simulink model "rocketmodel"  (R2019b)
settings: Solver=VariableStepAuto  StartTime=0.0  StopTime=1  RelTol=1e-3
values from neighbouring files (symbols this model uses):
  g = 9.8    [main_rocketmodel.m]    (also in main_sim_rocket.m; rocket_model.m; sim_lin.m; test_bangbang.m)
  gimbal_eq = 0    [main_rocketmodel.m]    (also in main_sim_rocket.m; sim_lin.m)
  J_T = 40267    [main_rocketmodel.m]    (also in main_sim_rocket.m; rocket_model.m = 10)
  K = minreal(Q/(1+Q*P))    [cost.m]    (also in cost_LQ.m = tf((conv(denQ{1},numK0{1})+conv(numQ{1},den_sys{1})),(conv(d; cost_con.m = tf((conv(denQ{1},numK0{1})+conv(numQ{1},den_sys{1})),(conv(d; cost_disturb.m = tf((conv(denQ{1},numK0{1})+conv(numQ{1},den_sys{1})),(conv(d; fminunc_LQ.m = tf((conv(denQ{1},numK0{1})+conv(numQ{1},den_sys{1})),(conv(d)
  K_2 = (tf((conv(denQ{1},num{1})+conv(numQ{1},den_sys{1})),(conv(denQ{1},den{1})-conv(numQ{1},num_sys{1}))))    [test.m]    (also in test_qvalues.m = Q_2/(1+Q_2*P))
  m = 549054    [main_rocketmodel.m]    (also in main_sim_rocket.m; rocket_model.m = 25.4; sim_lin.m; test_bangbang.m)
  sys = ss(A,B,C,D)    [controller_design.m]    (also in main_yp_fminunc.m; rocket_controllerdesign.m; rocket_controllerdesign_z.m; rocket_model.m)
  t_on = 14.6    [main_rocketmodel.m]    (also in main_sim_rocket.m; test_bangbang.m)
  Ts = 0.001    [main_rocketmodel.m]    (also in main_sim_rocket.m; sim_lin.m; square_sig.m; sum_squares_sig.m)
  x_0 = 0    [main_rocketmodel.m]    (also in main_sim_rocket.m)
  z_0 = 4000    [main_rocketmodel.m]    (also in main_sim_rocket.m; sim_lin.m; test_bangbang.m)
libraries: simulink x1
settings Model: Creator=bia  LastModifiedBy=bia
settings DataIOCC: ExternalInput=[t, Fe]  SignalLogging=off  DSMLogging=off

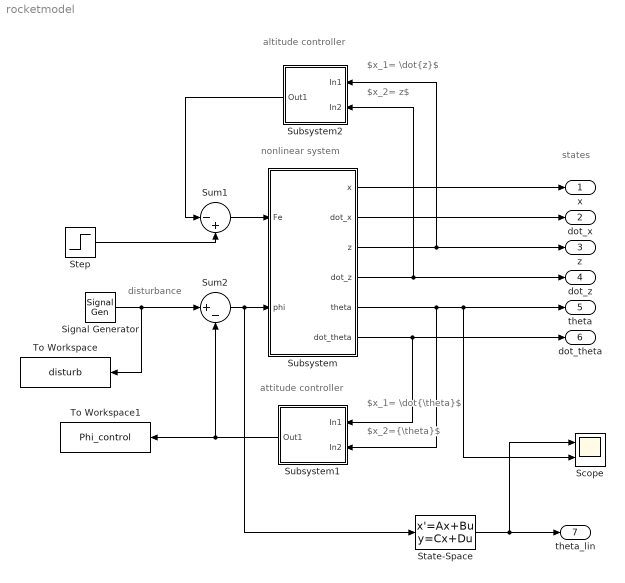
== system rocketmodel ==
  note: nonlinear system
  note: states
  note: $x_1= \dot{\theta}$
  note: $x_2={\theta}$
  note: attitude controller
  note: disturbance
  note: altitude controller
  note: $x_2= z$
  note: $x_1= \dot{z}$
  Scope : Scope  NumInputPorts=2
  Signal Generator : SignalGenerator  WaveForm=square  Amplitude=1e-6  Units=rad/sec
  State-Space : StateSpace  A=sys.A  B=sys.B  C=sys.C  D=sys.D  InitialCondition=0
  Step : Step  Time=t_on  Before=0.05*7e6  After=7e6  SampleTime=0
  Subsystem : Subsystem
  Subsystem1 : Subsystem
  Subsystem2 : Subsystem
  Sum1 : Sum  Inputs=|-+
  Sum2 : Sum  Inputs=|+-
  To Workspace : ToWorkspace  VariableName=disturb  SampleTime=Ts
  To Workspace1 : ToWorkspace  VariableName=Phi_control  SampleTime=Ts
  x : Outport
  "dot_x " : Outport  Port=2
  z : Outport  Port=3
  dot_z : Outport  Port=4
  theta : Outport  Port=5
  "dot_theta " : Outport  Port=6
  theta_lin : Outport  Port=7
  wires:
  Subsystem/1(x) -> x/1
  Subsystem/2(dot_x) -> "dot_x "/1
  Subsystem/4("dot_z ") -> dot_z/1, Subsystem2/2(In2)
  Sum2/1 -> State-Space/1, Subsystem/2(phi)
  Subsystem/3(z) -> z/1, Subsystem2/1(In1)
  Sum1/1 -> Subsystem/1(Fe)
  Step/1 -> Sum1/2
  Subsystem2/1(Out1) -> Sum1/1
  Subsystem/6("dot_theta ") -> Subsystem1/1(In1), "dot_theta "/1
  Subsystem/5(theta) -> Subsystem1/2(In2), Scope/2, theta/1
  Signal Generator/1 -> To Workspace/1, Sum2/1
  Subsystem1/1(Out1) -> To Workspace1/1, Sum2/2
  State-Space/1 -> Scope/1, theta_lin/1

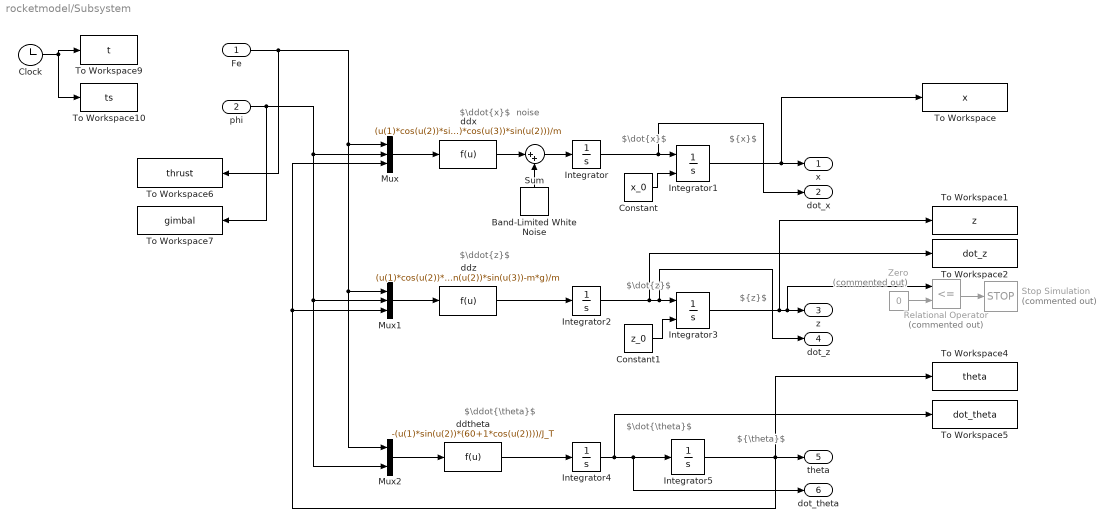
== system rocketmodel/Subsystem ==
  note: $\dot{z}$
  note: $\ddot{z}$
  note: ${z}$
  note: $\ddot{\theta}$
  note: $\ddot{x}$
  note: $\dot{x}$
  note: $\dot{\theta}$
  note: ${x}$
  note: ${\theta}$
  note: noise
  Fe : Inport
  phi : Inport  Port=2
  Band-Limited White Noise : simulink/Sources/Band-Limited White Noise  Cov=0  Ts=0.1  seed=[23341]
  Clock : Clock
  Constant : Constant  Value=x_0  SampleTime=Ts
  Constant1 : Constant  Value=z_0  SampleTime=Ts
  Integrator : Integrator  ContinuousStateAttributes='x_dot'
  Integrator1 : Integrator  InitialConditionSource=external  ContinuousStateAttributes='x'
  Integrator2 : Integrator  ContinuousStateAttributes='z_dot'
  Integrator3 : Integrator  InitialConditionSource=external  InitialCondition=50  LimitOutput=on  LowerSaturationLimit=0  ContinuousStateAttributes='z'
  Integrator4 : Integrator  ContinuousStateAttributes='theta_dot'
  Integrator5 : Integrator
  Mux : Mux  Inputs=3
  Mux1 : Mux  Inputs=3
  Mux2 : Mux  Inputs=2
  Relational Operator : RelationalOperator  Commented=on  Operator=<=  OutDataTypeStr=boolean  RndMeth=Nearest
  Stop Simulation : Stop  Commented=on
  Sum : Sum  Inputs=|++
  To Workspace : ToWorkspace  VariableName=x  SampleTime=Ts
  To Workspace1 : ToWorkspace  VariableName=z  SampleTime=Ts
  To Workspace10 : ToWorkspace  VariableName=ts  SampleTime=Ts
  To Workspace2 : ToWorkspace  VariableName=dot_z  SampleTime=Ts
  To Workspace4 : ToWorkspace  VariableName=theta  SampleTime=Ts
  To Workspace5 : ToWorkspace  VariableName=dot_theta  SampleTime=Ts
  To Workspace6 : ToWorkspace  VariableName=thrust  SampleTime=Ts
  To Workspace7 : ToWorkspace  VariableName=gimbal  SampleTime=Ts
  To Workspace9 : ToWorkspace  VariableName=t  SampleTime=-1
  Zero : Constant  Commented=on  Value=0  OutDataTypeStr=Inherit: Inherit via back propagation
  ddtheta : Fcn  Expr=-(u(1)*sin(u(2))*(60+1*cos(u(2))))/J_T
  ddx : Fcn  Expr=(u(1)*cos(u(2))*sin(u(3))+u(1)*cos(u(3))*sin(u(2)))/m
  ddz : Fcn  Expr=(u(1)*cos(u(2))*cos(u(3))-u(1)*sin(u(2))*sin(u(3))-m*g)/m
  x : Outport
  dot_x : Outport  Port=2
  z : Outport  Port=3
  "dot_z " : Outport  Port=4
  theta : Outport  Port=5
  "dot_theta " : Outport  Port=6
  wires:
  ddtheta/1 -> Integrator4/1
  Mux/1 -> ddx/1
  Integrator2/1 -> To Workspace2/1, "dot_z "/1, Integrator3/1
  Mux2/1 -> ddtheta/1
  Fe/1 -> To Workspace6/1, Mux2/1, Mux1/1, Mux/1
  Mux1/1 -> ddz/1
  Integrator/1 -> dot_x/1, Integrator1/1
  phi/1 -> To Workspace7/1, Mux2/2, Mux1/2, Mux/2
  Integrator3/1 -> z/1, Relational Operator/1, To Workspace1/1
  Integrator5/1 -> To Workspace4/1, Mux1/3, Mux/3, theta/1
  Constant1/1 -> Integrator3/2
  Constant/1 -> Integrator1/2
  Integrator4/1 -> Integrator5/1, "dot_theta "/1, To Workspace5/1
  Zero/1 -> Relational Operator/2
  Relational Operator/1 -> Stop Simulation/1
  Clock/1 -> To Workspace9/1, To Workspace10/1
  ddz/1 -> Integrator2/1
  Integrator1/1 -> To Workspace/1, x/1
  Band-Limited White Noise/1 -> Sum/2
  Sum/1 -> Integrator/1
  ddx/1 -> Sum/1

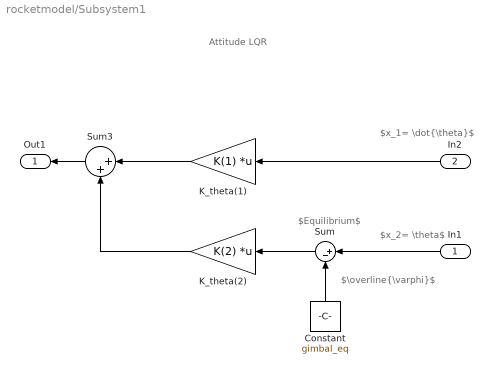
== system rocketmodel/Subsystem1 ==
  note: Attitude LQR
  note: $x_2= \theta$
  note: $x_1= \dot{\theta}$
  note: $Equilibrium$
  note: $\overline{\varphi}$
  In1 : Inport
  In2 : Inport  Port=2
  Constant : Constant  Value=gimbal_eq
  K_theta(1) : Gain  Gain=K(1)  Multiplication=Matrix(K*u)
  K_theta(2) : Gain  Gain=K(2)  Multiplication=Matrix(K*u)
  Sum : Sum  Inputs=|+-
  Sum3 : Sum  Inputs=|++
  Out1 : Outport
  wires:
  In1/1 -> Sum/1
  Sum3/1 -> Out1/1
  In2/1 -> K_theta(1)/1
  K_theta(2)/1 -> Sum3/2
  K_theta(1)/1 -> Sum3/1
  Sum/1 -> K_theta(2)/1
  Constant/1 -> Sum/2

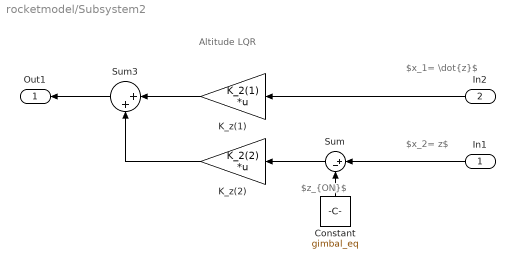
== system rocketmodel/Subsystem2 ==
  note: $x_1= \dot{z}$
  note: $x_2= z$
  note: Altitude LQR
  note: $z_{ON}$
  In1 : Inport
  In2 : Inport  Port=2
  Constant : Constant  Value=gimbal_eq
  K_z(1) : Gain  Gain=K_2(1)  Multiplication=Matrix(K*u)
  K_z(2) : Gain  Gain=K_2(2)  Multiplication=Matrix(K*u)
  Sum : Sum  Inputs=|+-
  Sum3 : Sum  Inputs=|++
  Out1 : Outport
  wires:
  In1/1 -> Sum/1
  In2/1 -> K_z(1)/1
  Sum/1 -> K_z(2)/1
  K_z(1)/1 -> Sum3/1
  K_z(2)/1 -> Sum3/2
  Sum3/1 -> Out1/1
  Constant/1 -> Sum/2
